simulink model "Joystick201401023GoldenTriangleLightTEST2"  (R2012b)
settings: Solver=ode4  StartTime=0.0  StopTime=inf  FixedStep=sample_time  RelTol=1e-3
InitFcn:
  | sample_time=0.005;%0.004;%0.0025;%0.02;
  | sample_time_Vicon = 0.005;
  | DeltaT = 0.02;
  | g = 9.81;
  | H0 = g%0.3165;
  | Kl = 1;
  | 
  | Omega_r = 1.31;%for Horizontal reference
  | Zeta_r = 1; %for Horizontal reference
  | Omega = 1.5;%1.31;%for Horizontal Control
  | Zeta = 0.5;    %for Horizontal Control
  | 
  | Omega_h_r = 2.2; %for vertical reference
  | Zeta_h_r = 1;  %for vertical reference
  | Omega_h = 2.2;    %for vertical control
  | Zeta_h = 1;         %for vertical control
  | PI=pi;
  | 
  | Mass = 1.1;
  | Acc_Max = 4;
  | Acc_Max_h = 4;
  | 
  | Max_RP = 60;
  | 
  | % for NN
  | n = 5;
  | r = 3;
  | n2 = 5;
  | NN_ST = 0.02;
  | 
  | GAMA_V = 3;
  | gama_V_e = 0.01;
  | 
  | GAMA_W = GAMA_V;
  | gama_W_e =0.01;
  | 
  | % deadzone
  | NN_Deadzone_Z = 0;
  | 
  | % inputs nomalizaton parameters
  | NN_Z_y_min = -3;
  | NN_Z_y_max = 0.5;
  | 
  | NN_Z_v_max = 8;
  | NN_Z_v_min = -NN_Z_v_max;
  | 
  | % alpha = 0.034;
  | alpha = 1;
  | % c_f = 0.0015;
  | c_f = 0.001;
  | c_y_tilt = 1*0.5;
  | 
  | %for WK paras
  | Heightcontrol = 0.08;
  | Scale_Factor=1;
  | yoffset=0;
  | 
  | load MaoBi_Oct04_2_int.mat
  | MB_Interp.time = [];
undefined symbols (not defined in the file or in its folder): DiscIntNeverNeededParam
libraries: simulink x8, X330_Control x4, vrlib x1
(part 1 of 2)
settings Model: Creator=ttcl3  LastModifiedBy=Vicon
settings SolverCC: MaxConsecutiveMinStep=auto
settings DataIOCC: SignalLoggingSaveFormat=ModelDataLogs
settings DebuggingCC: MultiTaskRateTransMsg=warning  FcnCallInpInsideContextMsg=UseLocalSettings
settings SFSimCC: SimParseCustomCode=off
settings GRTTargetCC: CombineOutputUpdateFcns=off  GRTInterface=on

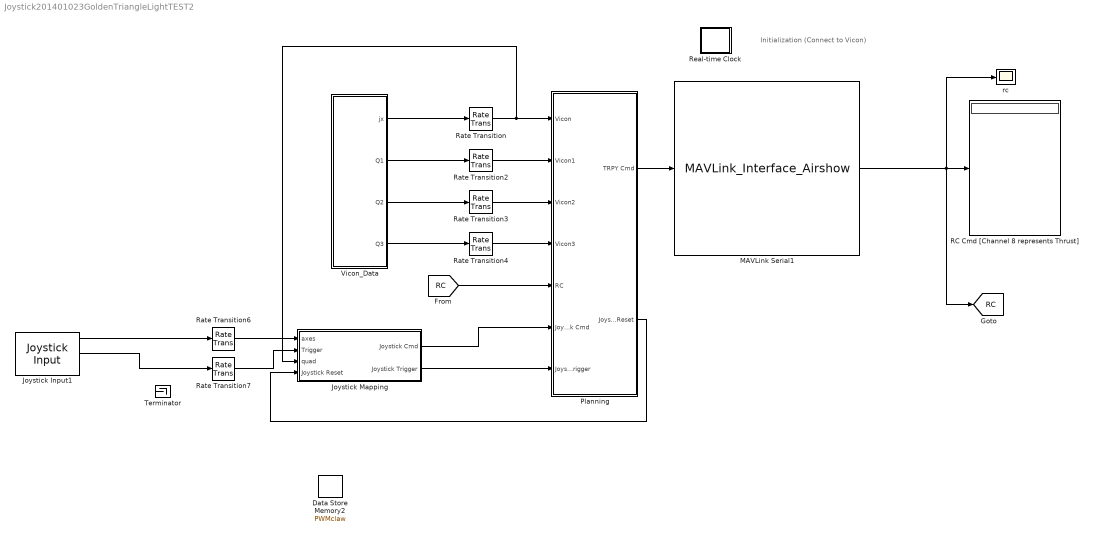
== system Joystick201401023GoldenTriangleLightTEST2 ==
  note: Initialization
      | (Connect to Vicon)
  Data Store Memory2 : DataStoreMemory  DataStoreName=PWMclaw  InitialValue=1690  OutDataTypeStr=double
  Joystick Input1 : vrlib/Joystick Input  joyid=1  adjustports=on  forcefeed=off
  Joystick Mapping : Subsystem
  MAVLink Serial1 : S-Function  FunctionName=MAVLink_Interface_Airshow  Parameters=COM_Port,Baud_Rate,MSG_INPUT,MSG_OUTPUT  EnableBusSupport=off  mask{COM_Port='COM2', Baud_Rate=57600, ATTITUDE_OUT=off, RC_SCALED=on, Quads_1=on, Quads_2=off, Quads_3=off, Quads_4=off, Quads_5=off, Quads_6=off}
      mask prompts: COM_Port "COM Port"; Baud_Rate "Baud Rate"; ATTITUDE_OUT "DEBUG"; RC_SCALED "RC CHANNELS SCALED"; Quads_1 "1 Quad"; Quads_2 "2 Quad"; Quads_3 "3 Quad"; Quads_4 "4 Quad"; Quads_5 "5 Quad"; Quads_6 "6 Quad"
      mask init:
      | MSG_ID_NUM_INPUT = [ uint8(221) uint8(222) uint8(223) uint8(224) uint8(225) uint8(226)];
      | MSG_ID_NAME_INPUT = [Quads_1 Quads_2 Quads_3 Quads_4 Quads_5 Quads_6];
      | 
      | MSG_ID_NUM_OUTPUT = [uint8(34) uint8(30)];
      | MSG_ID_NAME_OUTPUT = [RC_SCALED ATTITUDE_OUT ];
      | 
      | idx_input = find(MSG_ID_NAME_INPUT);
      | MSG_INPUT = MSG_ID_NUM_INPUT(idx_input);
      | 
      | idx_output = find(MSG_ID_NAME_OUTPUT);
      | MSG_OUTPUT = MSG_ID_NUM_OUTPUT(idx_output);
      mask Display:
      | % Block image
      | image(imread('10-inch Quad Heat Map.png'));
      | 
      | %Label block
      | fprintf('MAVLink Serial\n%s\n%dbps', COM_Port,  Baud_Rate)
      | 
      | 
      | %Label input ports
      | 
      | in = 1;
      | if (Quads_1 == 1)
      |     port_label('input', in, 'Quads_1');
      |     in = in + 1;
      | end
      | 
      | if (Quads_2 == 1)
      |     port_label('input', in, 'Quads_2');
      |     in = in + 1;
      | end
      | 
      | if (Quads_3 == 1)
      |     port_label('input', in, 'Quads_3');
      |     in = in + 1;
      | end
      | 
      | if (Quads_4 == 1)
      |     port_label('input', in, 'Quads_4');
      |     in = in + 1;
      | end
      | 
      | if (Quads_5 == 1)
      |     port_label('input', in, 'Quads_5');
      |     in = in + 1;
      | end
      | 
      | 
      | if (Quads_6 == 1)
      |     port_label('input', in, 'Quads_6');
      |     in = in + 1;
      | end
      | %Label output ports
      | 
      | out = 1;
      | if (RC_SCALED == 1)
      |     port_label('output', out, 'RC CMD');
      |     out = out + 1;
      | end
      | 
      | if (ATTITUDE_OUT == 1)
      |     port_label('output', out, 'DEBUG');
      |     out = out + 1;
      | end
  Planning : Subsystem
  RC Cmd [Channel 8 represents Thrust] : Display
  Rate Transition{,2..4,6..7} (6 alike) : RateTransition  OutPortSampleTime=0.02
  Real-time Clock : Subsystem  mask(Real-time Clock){sample_time=0.02, tolerance=1}
      mask prompts: sample_time "Synchronize with real-time every n seconds:"; tolerance "Real-time warning tolerance (seconds):"
      mask help: Real-time Synchronization Block
      mask Help: This block synchronizes simulation time with the PC real-time clock or UNIX system clock. The first dialog entry is the period at which the clock is checked to insure real-time synchronization. The second dialog entry is the number of seconds that the simulation time must be within real-time before a warning is printed.
      mask Display: plot(0,0,100,100,[40,60,60,54,54,64,69,76,82,77,81,83,83,81,78,74,70,64,57,49,41,35,32,30,30,31,34,40,47,47,40,40],[90,90,85,85,80,79,76,87,80,70,64,57,49,41,33,28,24,22,21,23,25,31,37,46,56,65,73,78,80,85,85,90],[69,53,53],[64,50,73])
  Terminator : Terminator
  Vicon_Data : Subsystem
  rc : Scope
      settings: TimeRange=10  YMin=-1  YMax=0.1
  tag scope: RC=global
  wires:
  [RC] -> Planning/5(RC)
  MAVLink Serial1/1 -> [RC], rc/1, RC Cmd [Channel 8 represents Thrust]/1
  Rate Transition/1 -> Joystick Mapping/3(quad), Planning/1(Vicon)
  Vicon_Data/4(Q3) -> Rate Transition4/1
  Vicon_Data/3(Q2) -> Rate Transition3/1
  Vicon_Data/2(Q1) -> Rate Transition2/1
  Rate Transition4/1 -> Planning/4(Vicon3)
  Rate Transition3/1 -> Planning/3(Vicon2)
  Rate Transition2/1 -> Planning/2(Vicon1)
  Planning/1(TRPY Cmd) -> MAVLink Serial1/1
  Joystick Input1/1 -> Rate Transition6/1
  Joystick Mapping/1(Joystick Cmd) -> Planning/6(Joystick Cmd)
  Rate Transition6/1 -> Joystick Mapping/1(axes)
  Rate Transition7/1 -> Joystick Mapping/2(Trigger)
  Vicon_Data/1(jx) -> Rate Transition/1
  Planning/2(JoystickReset) -> Joystick Mapping/4(Joystick Reset)
  Joystick Mapping/2(Joystick Trigger) -> Planning/7(Joystick Trigger)
  Joystick Input1/2 -> Rate Transition7/1
  ? -> Terminator/1

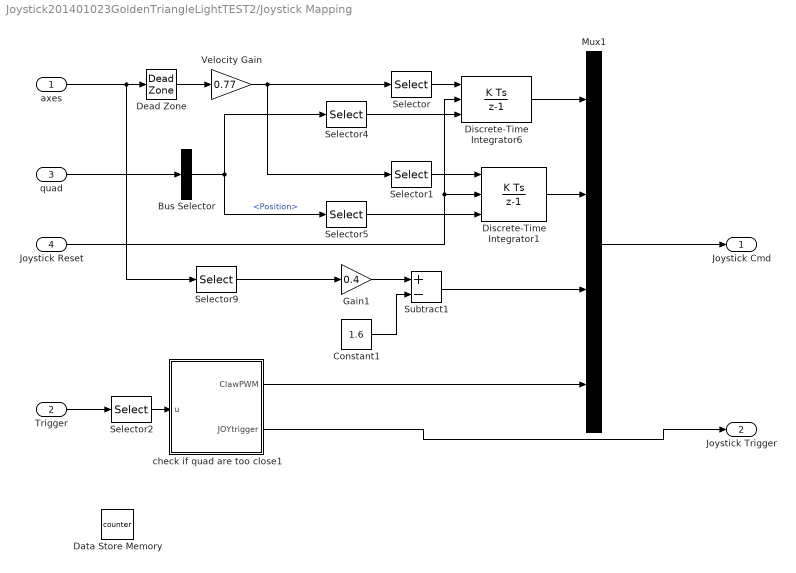
== system Joystick201401023GoldenTriangleLightTEST2/Joystick Mapping ==
  axes : Inport
  Trigger : Inport  Port=2
  quad : Inport  Port=3
  Joystick Reset : Inport  Port=4
  Bus Selector : BusSelector  OutputSignals=Position
  Constant1 : Constant  Value=1.6
  Data Store Memory : DataStoreMemory  DataStoreName=counter  InitialValue=25  OutDataTypeStr=double
  Dead Zone : DeadZone  LowerValue=-0.01  UpperValue=0.01  SaturateOnIntegerOverflow=on
  Discrete-Time Integrator1 : DiscreteIntegrator  gainval=1  ExternalReset=level  InitialConditionSource=external  SampleTime=0.02  OutMin=-3.5  OutMax=3.5  LimitOutput=on  UpperSaturationLimit=3.5  LowerSaturationLimit=-3.5  ICPrevOutput=DiscIntNeverNeededParam  ICPrevScaledInput=DiscIntNeverNeededParam
  Discrete-Time Integrator6 : DiscreteIntegrator  gainval=1  ExternalReset=level  InitialConditionSource=external  SampleTime=0.02  OutMin=-3.5  OutMax=3.5  LimitOutput=on  UpperSaturationLimit=3.5  LowerSaturationLimit=-3.5  ICPrevOutput=DiscIntNeverNeededParam  ICPrevScaledInput=DiscIntNeverNeededParam
  Gain1 : Gain  Gain=0.4
  Mux1 : Mux
  Selector : Selector  IndexOptions=Index vector (dialog)  Indices=[1]  OutputSizes=1
  Selector1 : Selector  IndexOptions=Index vector (dialog)  Indices=[2]  OutputSizes=1
  Selector2 : Selector  IndexOptions=Index vector (dialog)  Indices=[1]  OutputSizes=1
  Selector4 : Selector  InputPortWidth=3  IndexOptions=Index vector (dialog)  Indices=[1]  OutputSizes=1
  Selector5 : Selector  InputPortWidth=3  IndexOptions=Index vector (dialog)  Indices=[2]  OutputSizes=1
  Selector9 : Selector  IndexOptions=Index vector (dialog)  Indices=[3]  OutputSizes=1
  Subtract1 : Sum  Inputs=+-  OutMin=-2.5  OutMax=-1
  Velocity Gain : Gain  Gain=0.77
  check if quad are too close1 : MATLAB Function  TreatAsAtomicUnit=on
  Joystick Cmd : Outport
  Joystick Trigger : Outport  Port=2
  wires:
  Selector1/1 -> Discrete-Time Integrator1/1
  Selector/1 -> Discrete-Time Integrator6/1
  Velocity Gain/1 -> Selector1/1, Selector/1
  axes/1 -> Dead Zone/1, Selector9/1
  Discrete-Time Integrator6/1 -> Mux1/1
  Discrete-Time Integrator1/1 -> Mux1/2
  Mux1/1 -> Joystick Cmd/1
  check if quad are too close1/1(ClawPWM) -> Mux1/4
  Selector2/1 -> check if quad are too close1/1(u)
  Trigger/1 -> Selector2/1
  quad/1 -> Bus Selector/1
  Bus Selector/1 -> Selector4/1, Selector5/1  "<Position>"
  Selector4/1 -> Discrete-Time Integrator6/3
  Selector5/1 -> Discrete-Time Integrator1/3
  Joystick Reset/1 -> Discrete-Time Integrator1/2, Discrete-Time Integrator6/2
  check if quad are too close1/2(JOYtrigger) -> Joystick Trigger/1
  Constant1/1 -> Subtract1/2
  Selector9/1 -> Gain1/1
  Gain1/1 -> Subtract1/1
  Subtract1/1 -> Mux1/3
  Dead Zone/1 -> Velocity Gain/1

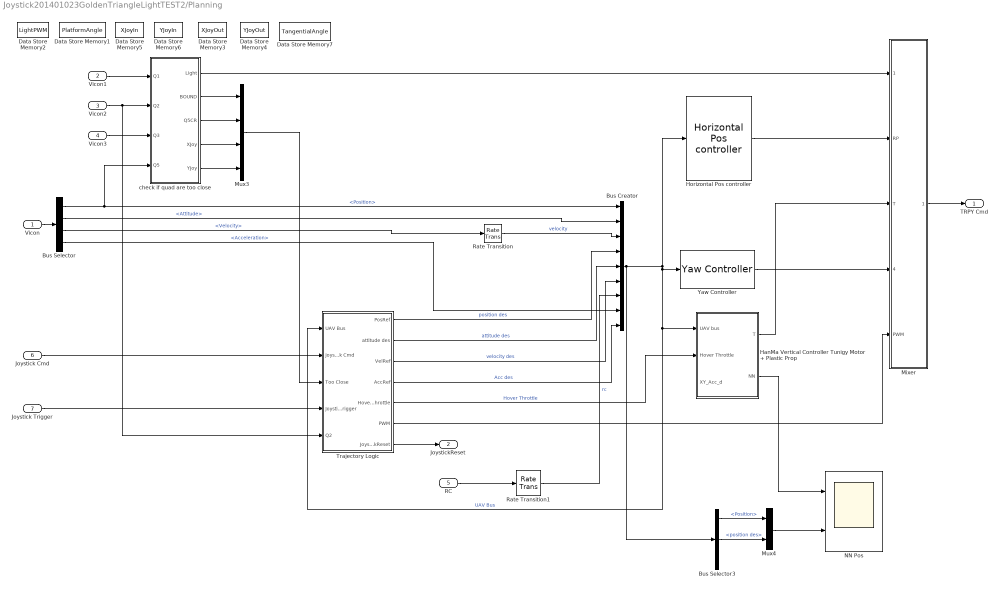
== system Joystick201401023GoldenTriangleLightTEST2/Planning ==
  Vicon : Inport
  Vicon1 : Inport  Port=2
  Vicon2 : Inport  Port=3
  Vicon3 : Inport  Port=4
  RC : Inport  Port=5
  Joystick Cmd : Inport  Port=6
  Joystick Trigger : Inport  Port=7
  Bus Creator : BusCreator  Inputs=9
  Bus Selector : BusSelector  OutputSignals=Position,Attitude,Velocity,Acceleration
  Bus Selector3 : BusSelector  OutputSignals=Position,position des,Attitude
  Data Store Memory1 : DataStoreMemory  DataStoreName=PlatformAngle  OutDataTypeStr=double
  Data Store Memory2 : DataStoreMemory  DataStoreName=LightPWM  OutMin=-3.3  OutMax=3.3  OutDataTypeStr=double
  Data Store Memory3 : DataStoreMemory  DataStoreName=XJoyOut  OutMin=-3.5  OutMax=3.5  OutDataTypeStr=double
  Data Store Memory4 : DataStoreMemory  DataStoreName=YJoyOut  OutMin=-3.5  OutMax=3.5  OutDataTypeStr=double
  Data Store Memory5 : DataStoreMemory  DataStoreName=XJoyIn  OutMin=-3.3  OutMax=3.3  OutDataTypeStr=double
  Data Store Memory6 : DataStoreMemory  DataStoreName=YJoyIn  OutMin=-3.3  OutMax=3.3  OutDataTypeStr=double
  Data Store Memory7 : DataStoreMemory  DataStoreName=TangentialAngle  OutDataTypeStr=double
  HanMa Vertical Controller Tunigy Motor + Plastic Prop : Subsystem  mask{Omega_h=Omega_h, Zeta_h=Zeta_h, PID_I_h=0, mass=1.1}
      mask prompts: Omega_h "Omega (P Gain  = Omega^2)"; Zeta_h "Zeta (D Gain = 2*Omega*Zeta)"; PID_I_h "I Gain"
  Horizontal Pos controller : X330_Control/Horizontal Pos controller  Max_RP=Max_RP  Omega=Omega  PID_i=0.5  Zeta=Zeta
      link override Horizontal Position Controller/Saturation1: UpperLimit=3.4  LowerLimit=-3.4
  Mixer : Subsystem
  Mux3 : Mux
  Mux4 : Mux  Inputs=2
  NN Pos : Scope  NumInputPorts=2
      settings: TimeRange=90  YMin=-1.25~-3  YMax=3.5~0  SaveName=ScopeData3
  Rate Transition : RateTransition  OutPortSampleTime=0.02
  Rate Transition1 : RateTransition  OutPortSampleTime=0.02
  Trajectory Logic : Subsystem
  Yaw Controller : X330_Control/Yaw Controller
  check if quad are too close : MATLAB Function  TreatAsAtomicUnit=on
  TRPY Cmd : Outport
  JoystickReset : Outport  Port=2
  wires:
  Horizontal Pos controller/1 -> Mixer/2(RP)
  Rate Transition/1 -> Bus Creator/3  "velocity"
  Rate Transition1/1 -> Bus Creator/7  "rc"
  Bus Creator/1 -> Yaw Controller/1, Trajectory Logic/1(UAV Bus), HanMa Vertical Controller Tunigy Motor + Plastic Prop/1(UAV bus), Horizontal Pos controller/1, Bus Selector3/1  "UAV Bus"
  Yaw Controller/1 -> Mixer/4(Yaw rate)
  HanMa Vertical Controller Tunigy Motor + Plastic Prop/1(T) -> Mixer/3(T)
  Bus Selector/4 -> Bus Creator/8  "<Acceleration>"
  Trajectory Logic/1(PosRef) -> Bus Creator/4  "position des"
  Trajectory Logic/2(attitude des) -> Bus Creator/5  "attitude des"
  Trajectory Logic/3(VelRef) -> Bus Creator/6  "velocity des"
  Trajectory Logic/5(HoverThrottle) -> HanMa Vertical Controller Tunigy Motor + Plastic Prop/2(Hover Throttle)  "Hover Throttle"
  Bus Selector/1 -> check if quad are too close/4(Q5), Bus Creator/1  "<Position>"
  Bus Selector/2 -> Bus Creator/2  "<Attitude>"
  Bus Selector/3 -> Rate Transition/1  "<Velocity>"
  Vicon/1 -> Bus Selector/1
  Mixer/1(XYZ RPY) -> TRPY Cmd/1
  Trajectory Logic/4(AccRef) -> Bus Creator/9  "Acc des"
  RC/1 -> Rate Transition1/1
  Trajectory Logic/6(PWM) -> Mixer/5(PWM)
  Mux4/1 -> NN Pos/2
  Bus Selector3/1 -> Mux4/1  "<Position>"
  Bus Selector3/2 -> Mux4/2  "<position des>"
  HanMa Vertical Controller Tunigy Motor + Plastic Prop/2(NN) -> NN Pos/1
  Joystick Cmd/1 -> Trajectory Logic/2(Joystick Cmd)
  Mux3/1 -> Trajectory Logic/3(Too Close)
  Vicon3/1 -> check if quad are too close/3(Q3)
  Vicon2/1 -> Trajectory Logic/5(Q2), check if quad are too close/2(Q2)
  Vicon1/1 -> check if quad are too close/1(Q1)
  Trajectory Logic/7(JoystickReset) -> JoystickReset/1
  check if quad are too close/2(BOUND) -> Mux3/1
  check if quad are too close/3(Q5CR) -> Mux3/2
  check if quad are too close/4(XJoy) -> Mux3/3
  check if quad are too close/5(YJoy) -> Mux3/4
  Joystick Trigger/1 -> Trajectory Logic/4(Joystick Trigger)
  check if quad are too close/1(Light) -> Mixer/1(Light PWM)

== system Joystick201401023GoldenTriangleLightTEST2/Real-time Clock ==
  Real-time Clock : S-Function  FunctionName=rtclock  Parameters=sample_time, tolerance  EnableBusSupport=off

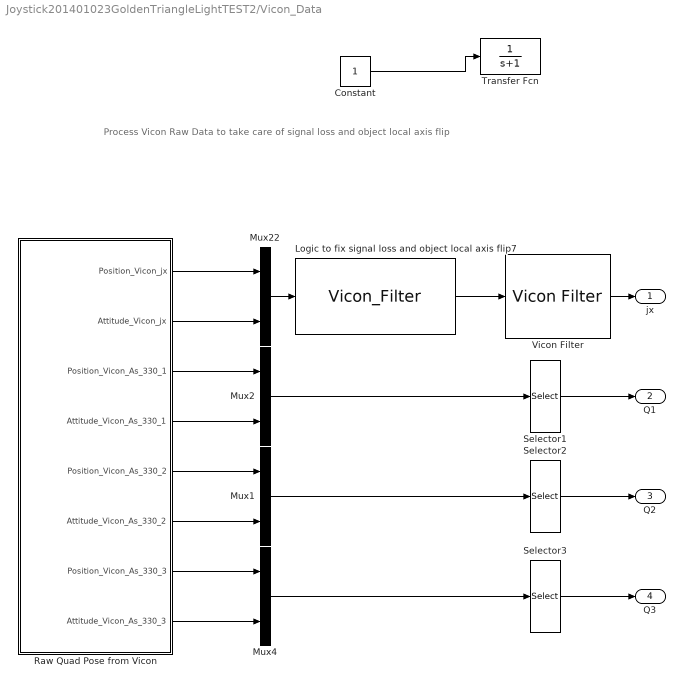
== system Joystick201401023GoldenTriangleLightTEST2/Vicon_Data ==
  note: Process Vicon Raw Data to take care of signal loss and object local axis flip
  Constant : Constant
  Logic to fix signal loss and object local axis flip7 : M-S-Function  FunctionName=Vicon_Filter
  Mux{1..2,4,22} (4 alike) : Mux  Inputs=2
  Raw Quad Pose from Vicon : Subsystem
  Selector1 : Selector  InputPortWidth=6  IndexOptions=Index vector (dialog)  Indices=[1 2]  OutputSizes=1
  Selector2 : Selector  InputPortWidth=6  IndexOptions=Index vector (dialog)  Indices=[1 2 3]  OutputSizes=1
  Selector3 : Selector  InputPortWidth=6  IndexOptions=Index vector (dialog)  Indices=[1 2]  OutputSizes=1
  Transfer Fcn : TransferFcn  Denominator=[1 1]
  Vicon Filter : X330_Control/Vicon Filter
  jx : Outport
  Q1 : Outport  Port=2
  Q2 : Outport  Port=3
  Q3 : Outport  Port=4
  wires:
  Raw Quad Pose from Vicon/2(Attitude_Vicon_jx) -> Mux22/2
  Raw Quad Pose from Vicon/1(Position_Vicon_jx) -> Mux22/1
  Logic to fix signal loss and object local axis flip7/1 -> Vicon Filter/1
  Mux2/1 -> Selector1/1
  Selector1/1 -> Q1/1
  Raw Quad Pose from Vicon/4(Attitude_Vicon_As_330_1) -> Mux2/2
  Raw Quad Pose from Vicon/3(Position_Vicon_As_330_1) -> Mux2/1
  Selector2/1 -> Q2/1
  Mux1/1 -> Selector2/1
  Raw Quad Pose from Vicon/5(Position_Vicon_As_330_2) -> Mux1/1
  Raw Quad Pose from Vicon/6(Attitude_Vicon_As_330_2) -> Mux1/2
  Mux4/1 -> Selector3/1
  Selector3/1 -> Q3/1
  Raw Quad Pose from Vicon/8(Attitude_Vicon_As_330_3) -> Mux4/2
  Raw Quad Pose from Vicon/7(Position_Vicon_As_330_3) -> Mux4/1
  Constant/1 -> Transfer Fcn/1
  Mux22/1 -> Logic to fix signal loss and object local axis flip7/1
  Vicon Filter/1 -> jx/1

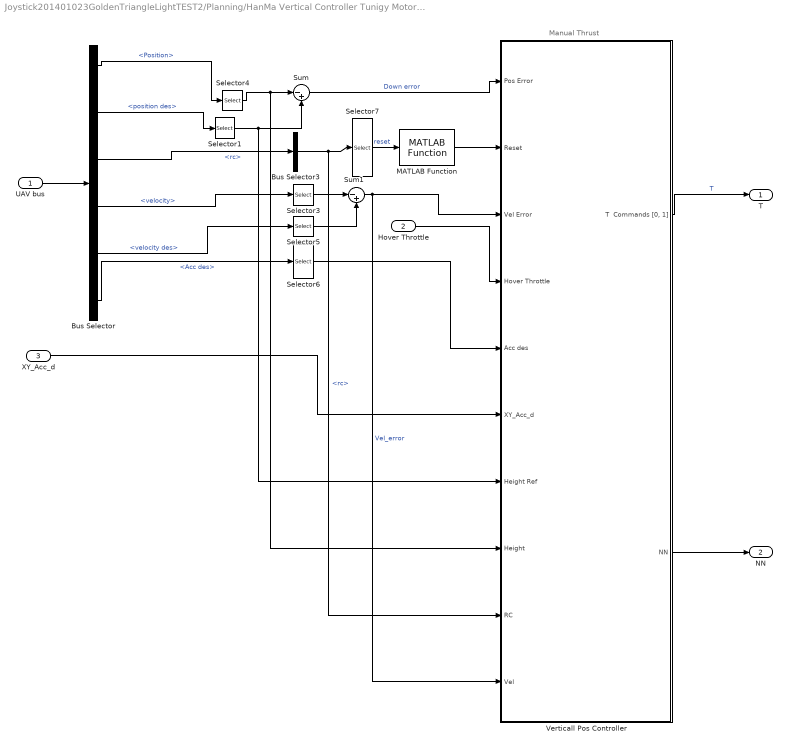
== system Joystick201401023GoldenTriangleLightTEST2/Planning/HanMa Vertical Controller Tunigy Motor + Plastic Prop ==
  note: Manual Thrust
  UAV bus : Inport
  Hover Throttle : Inport  Port=2
  XY_Acc_d : Inport  Port=3
  Bus Selector : BusSelector  OutputSignals=Position,position des,rc,velocity,velocity des,Acc des
  Bus Selector3 : BusSelector  OutputSignals=rc
  MATLAB Function : X330_Control/NN For Height AxiMotor + APC Prop/MATLAB Function
  Selector{1,3..5} (4 alike) : Selector  InputPortWidth=3  IndexOptions=Index vector (dialog)  Indices=[3]  OutputSizes=1
  Selector6 : Selector  InputPortWidth=4  IndexOptions=Index vector (dialog)  Indices=[3]  OutputSizes=1
  Selector7 : Selector  InputPortWidth=8  IndexOptions=Index vector (dialog)  Indices=[7]  OutputSizes=1
  Sum : Sum  Inputs=|-+
  Sum1 : Sum  Inputs=|-+
  Verticall Pos Controller : Subsystem
  T : Outport
  NN : Outport  Port=2
  wires:
  XY_Acc_d/1 -> Verticall Pos Controller/6(XY_Acc_d)
  Verticall Pos Controller/1("T  Commands [0, 1]") -> T/1  "T"
  Selector6/1 -> Verticall Pos Controller/5(Acc des)
  Bus Selector/6 -> Selector6/1  "<Acc des>"
  Hover Throttle/1 -> Verticall Pos Controller/4(Hover Throttle)
  Bus Selector/5 -> Selector5/1  "<velocity des>"
  Bus Selector/4 -> Selector3/1  "<velocity>"
  Selector5/1 -> Sum1/2
  Selector3/1 -> Sum1/1
  Sum1/1 -> Verticall Pos Controller/3(Vel Error), Verticall Pos Controller/10(Vel)  "Vel_error"
  Selector7/1 -> MATLAB Function/1  "reset"
  Bus Selector3/1 -> Selector7/1, Verticall Pos Controller/9(RC)  "<rc>"
  Selector1/1 -> Sum/2, Verticall Pos Controller/7(Height Ref)
  Selector4/1 -> Sum/1, Verticall Pos Controller/8(Height)
  Sum/1 -> Verticall Pos Controller/1(Pos Error)  "Down error"
  Bus Selector/2 -> Selector1/1  "<position des>"
  Bus Selector/1 -> Selector4/1  "<Position>"
  Bus Selector/3 -> Bus Selector3/1  "<rc>"
  UAV bus/1 -> Bus Selector/1
  Verticall Pos Controller/2(NN) -> NN/1
  MATLAB Function/1 -> Verticall Pos Controller/2(Reset)

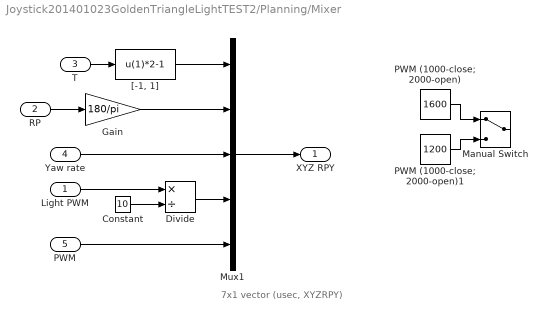
== system Joystick201401023GoldenTriangleLightTEST2/Planning/Mixer ==
  note: 7x1 vector (usec, XYZRPY)
  Light PWM : Inport
  RP : Inport  Port=2
  T : Inport  Port=3
  Yaw rate : Inport  Port=4
  PWM : Inport  Port=5
  Constant : Constant  Value=10
  Divide : Product  Inputs=*/
  Gain : Gain  Gain=180/pi
  Manual Switch : ManualSwitch
  Mux1 : Mux  Inputs=5
  PWM (1000-close; 2000-open) : Constant  Value=1600  SampleTime=0.02
  PWM (1000-close; 2000-open)1 : Constant  Value=1200  SampleTime=0.02
  "[-1, 1]" : Fcn  Expr=u(1)*2-1
  XYZ RPY : Outport
  wires:
  Mux1/1 -> XYZ RPY/1
  T/1 -> "[-1, 1]"/1
  RP/1 -> Gain/1
  PWM (1000-close; 2000-open)/1 -> Manual Switch/1
  PWM (1000-close; 2000-open)1/1 -> Manual Switch/2
  Gain/1 -> Mux1/2
  "[-1, 1]"/1 -> Mux1/1
  PWM/1 -> Mux1/5
  Constant/1 -> Divide/2
  Yaw rate/1 -> Mux1/3
  Divide/1 -> Mux1/4
  Light PWM/1 -> Divide/1

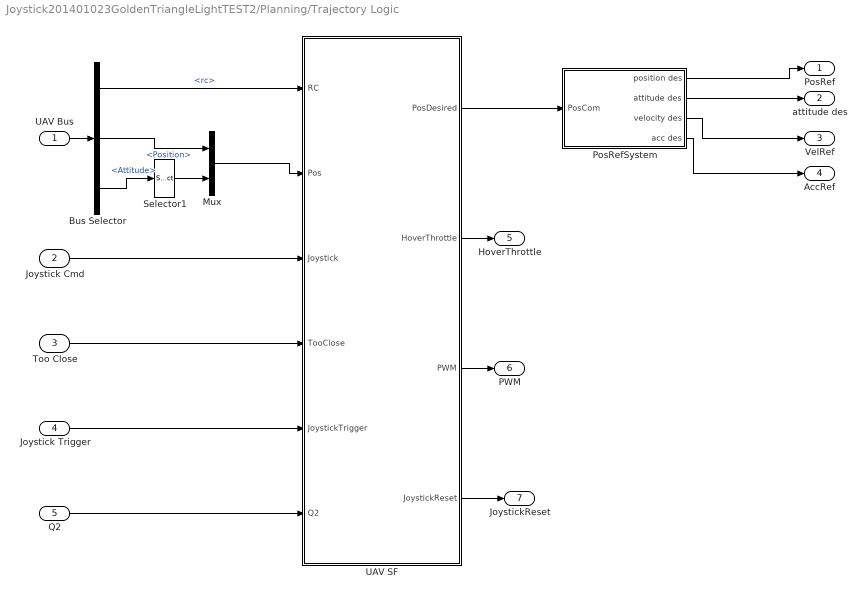
== system Joystick201401023GoldenTriangleLightTEST2/Planning/Trajectory Logic ==
  UAV Bus : Inport
  Joystick Cmd : Inport  Port=2
  Too Close : Inport  Port=3
  Joystick Trigger : Inport  Port=4
  Q2 : Inport  Port=5
  Bus Selector : BusSelector  OutputSignals=rc,Position,Attitude
  Mux : Mux  Inputs=2
  PosRefSystem : Subsystem  AncestorBlock=X330_Control/PosRefSystem  mask{Omega_r=Omega_r, Zeta_r=Zeta_r, Acc_Max=Acc_Max, Omega_h_r=Omega_h_r, Zeta_h_r=Zeta_h_r, Acc_h_Max=Acc_Max_h}
      mask prompts: Omega_r "Omega_r (P Gain= Omega_r^2)"; Zeta_r "Zeta_r (D = 2*Omega_r*Zeta_r)"
  Selector1 : Selector  InputPortWidth=3  IndexOptions=Index vector (dialog)  Indices=[3]  OutputSizes=1
  UAV SF : Stateflow chart  TreatAsAtomicUnit=on
  PosRef : Outport
  attitude des : Outport  Port=2
  VelRef : Outport  Port=3
  AccRef : Outport  Port=4
  HoverThrottle : Outport  Port=5
  PWM : Outport  Port=6
  JoystickReset : Outport  Port=7
  wires:
  UAV SF/1(PosDesired) -> PosRefSystem/1(PosCom)
  Bus Selector/1 -> UAV SF/1(RC)  "<rc>"
  UAV SF/2(HoverThrottle) -> HoverThrottle/1
  UAV Bus/1 -> Bus Selector/1
  Bus Selector/2 -> Mux/1  "<Position>"
  Bus Selector/3 -> Selector1/1  "<Attitude>"
  Selector1/1 -> Mux/2
  Mux/1 -> UAV SF/2(Pos)
  UAV SF/3(PWM) -> PWM/1
  PosRefSystem/1(position des) -> PosRef/1
  PosRefSystem/3(velocity des) -> VelRef/1
  PosRefSystem/4(acc des) -> AccRef/1
  PosRefSystem/2(attitude des) -> attitude des/1
  Joystick Cmd/1 -> UAV SF/3(Joystick)
  Too Close/1 -> UAV SF/4(TooClose)
  UAV SF/4(JoystickReset) -> JoystickReset/1
  Joystick Trigger/1 -> UAV SF/5(JoystickTrigger)
  Q2/1 -> UAV SF/6(Q2)

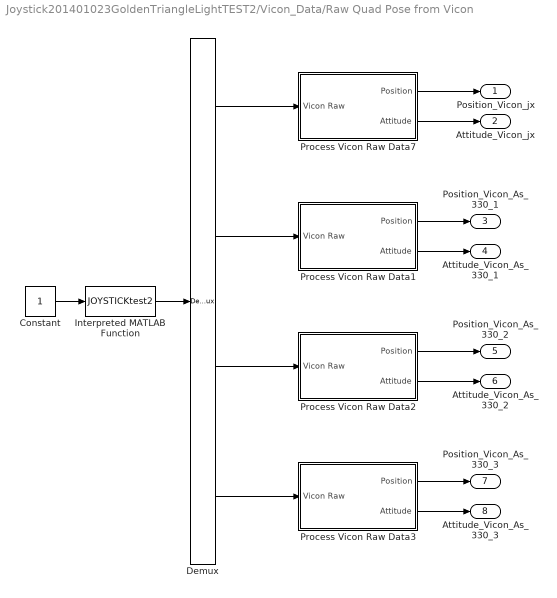
== system Joystick201401023GoldenTriangleLightTEST2/Vicon_Data/Raw Quad Pose from Vicon ==
  Constant : Constant
  Demux : Demux
  Interpreted MATLAB Function : MATLABFcn  MATLABFcn=JOYSTICKtest2  SampleTime=0.005
  Process Vicon Raw Data1 : Subsystem
  Process Vicon Raw Data2 : Subsystem
  Process Vicon Raw Data3 : Subsystem
  Process Vicon Raw Data7 : Subsystem
  Position_Vicon_jx : Outport
  Attitude_Vicon_jx : Outport  Port=2
  Position_Vicon_As_330_1 : Outport  Port=3
  Attitude_Vicon_As_330_1 : Outport  Port=4
  Position_Vicon_As_330_2 : Outport  Port=5
  Attitude_Vicon_As_330_2 : Outport  Port=6
  Position_Vicon_As_330_3 : Outport  Port=7
  Attitude_Vicon_As_330_3 : Outport  Port=8
  wires:
  Process Vicon Raw Data7/1(Position) -> Position_Vicon_jx/1
  Process Vicon Raw Data7/2(Attitude) -> Attitude_Vicon_jx/1
  Constant/1 -> Interpreted MATLAB Function/1
  Interpreted MATLAB Function/1 -> Demux/1
  Process Vicon Raw Data1/1(Position) -> Position_Vicon_As_330_1/1
  Process Vicon Raw Data1/2(Attitude) -> Attitude_Vicon_As_330_1/1
  Process Vicon Raw Data2/1(Position) -> Position_Vicon_As_330_2/1
  Process Vicon Raw Data2/2(Attitude) -> Attitude_Vicon_As_330_2/1
  Process Vicon Raw Data3/1(Position) -> Position_Vicon_As_330_3/1
  Process Vicon Raw Data3/2(Attitude) -> Attitude_Vicon_As_330_3/1
  Demux/1 -> Process Vicon Raw Data7/1(Vicon Raw)
  Demux/2 -> Process Vicon Raw Data1/1(Vicon Raw)
  Demux/3 -> Process Vicon Raw Data2/1(Vicon Raw)
  Demux/4 -> Process Vicon Raw Data3/1(Vicon Raw)

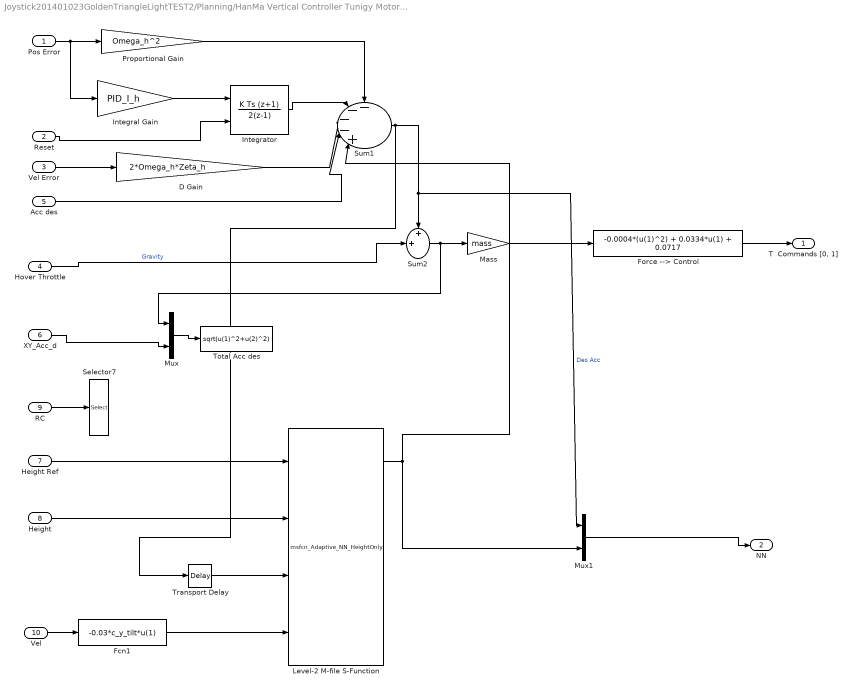
== system Joystick201401023GoldenTriangleLightTEST2/Planning/HanMa Vertical Controller Tunigy Motor + Plastic Prop/Verticall Pos Controller ==
  Pos Error : Inport
  Reset : Inport  Port=2
  Vel Error : Inport  Port=3
  Hover Throttle : Inport  Port=4
  Acc des : Inport  Port=5
  XY_Acc_d : Inport  Port=6
  Height Ref : Inport  Port=7
  Height : Inport  Port=8
  RC : Inport  Port=9
  Vel : Inport  Port=10
  D Gain : Gain  Gain=2*Omega_h*Zeta_h  OutDataTypeStr=double
  Fcn1 : Fcn  Expr=-0.03*c_y_tilt*u(1)
  Force --> Control : Fcn  Expr=-0.0004*(u(1)^2) + 0.0334*u(1) + 0.0717
  Integral Gain : Gain  DisableCoverage=on  Gain=PID_I_h  ParamDataTypeStr=double  OutDataTypeStr=double
  Integrator : DiscreteIntegrator  DisableCoverage=on  IntegratorMethod=Integration: Trapezoidal  ExternalReset=level  InitialConditionMode=State only (most efficient)  SampleTime=-1  OutDataTypeStr=double  UpperSaturationLimit=0.3  LowerSaturationLimit=-0.3  ICPrevOutput=DiscIntNeverNeededParam  ICPrevScaledInput=DiscIntNeverNeededParam
  Level-2 M-file S-Function : M-S-Function  FunctionName=msfcn_Adaptive_NN_HeightOnly  Parameters=n,r,n2,NN_ST,GAMA_V,gama_V_e,GAMA_W,gama_W_e,alpha,c_f,c_y_tilt,NN_Deadzone_Z,NN_Z_y_min,NN_Z_y_max,NN_Z_v_min,NN_Z_v_max
      mask Display: fprintf('Output Feedback NN \n Control Block')
  Mass : Gain  DisableCoverage=on  Gain=mass  ParamDataTypeStr=double  OutDataTypeStr=double
  Mux : Mux  Inputs=2
  Mux1 : Mux  Inputs=2
  Proportional Gain : Gain  DisableCoverage=on  Gain=Omega_h^2  ParamDataTypeStr=double  OutDataTypeStr=double
  Selector7 : Selector  InputPortWidth=8  IndexOptions=Index vector (dialog)  Indices=[6]  OutputSizes=1
  Sum1 : Sum  DisableCoverage=on  Inputs=----+|  AccumDataTypeStr=double  OutDataTypeStr=double  SampleTime=0.02
  Sum2 : Sum  DisableCoverage=on  Inputs=++|  AccumDataTypeStr=double  OutDataTypeStr=double  SampleTime=0.02
  Total Acc des : Fcn  Expr=sqrt(u(1)^2+u(2)^2)
  Transport Delay : TransportDelay  DelayTime=0.02
  "T  Commands [0, 1]" : Outport
  NN : Outport  Port=2
  wires:
  Force --> Control/1 -> "T  Commands [0, 1]"/1
  Sum2/1 -> Mux/1, Mass/1
  XY_Acc_d/1 -> Mux/2
  Mux/1 -> Total Acc des/1
  Mass/1 -> Force --> Control/1
  Sum1/1 -> Transport Delay/1, Sum2/1, Mux1/1  "Des Acc"
  Hover Throttle/1 -> Sum2/2  "Gravity"
  Acc des/1 -> Sum1/4
  D Gain/1 -> Sum1/3
  Vel Error/1 -> D Gain/1
  Reset/1 -> Integrator/2
  Pos Error/1 -> Integral Gain/1, Proportional Gain/1
  Proportional Gain/1 -> Sum1/1
  Integrator/1 -> Sum1/2
  Integral Gain/1 -> Integrator/1
  Height Ref/1 -> Level-2 M-file S-Function/1
  Level-2 M-file S-Function/1 -> Mux1/2, Sum1/5
  RC/1 -> Selector7/1
  Fcn1/1 -> Level-2 M-file S-Function/4
  Transport Delay/1 -> Level-2 M-file S-Function/3
  Mux1/1 -> NN/1
  Vel/1 -> Fcn1/1
  Height/1 -> Level-2 M-file S-Function/2

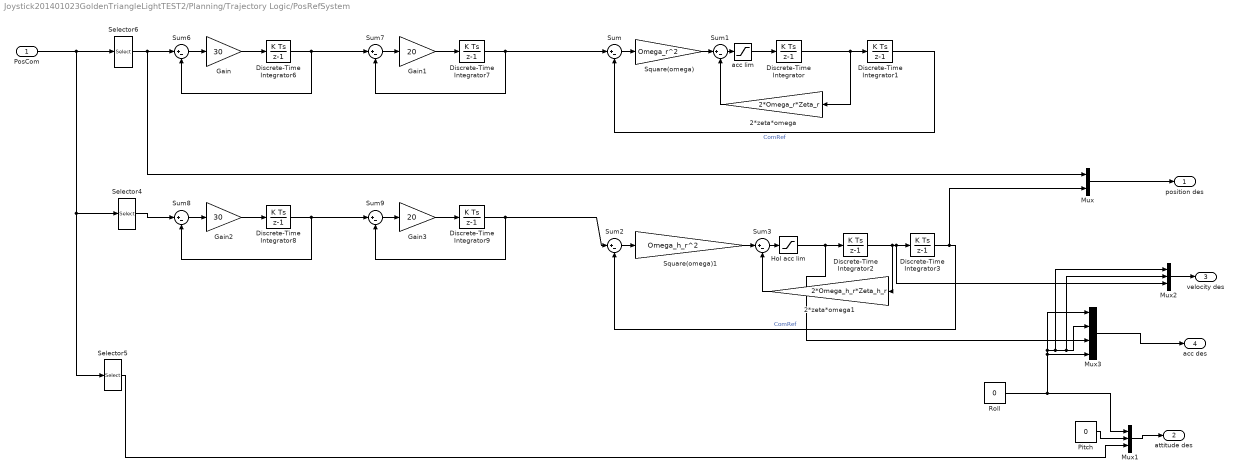
== system Joystick201401023GoldenTriangleLightTEST2/Planning/Trajectory Logic/PosRefSystem ==
  PosCom : Inport
  2*zeta*omega : Gain  Gain=2*Omega_r*Zeta_r
  2*zeta*omega1 : Gain  Gain=2*Omega_h_r*Zeta_h_r
  Discrete-Time Integrator{,1..3,6..9} (8 alike) : DiscreteIntegrator  SampleTime=-1  ICPrevOutput=DiscIntNeverNeededParam  ICPrevScaledInput=DiscIntNeverNeededParam
  Gain : Gain  Gain=30
  Gain1 : Gain  Gain=20
  Gain2 : Gain  Gain=30
  Gain3 : Gain  Gain=20
  Hol acc lim : Saturate  UpperLimit=Acc_h_Max  LowerLimit=-Acc_h_Max
  Mux : Mux  Inputs=2
  Mux1 : Mux  Inputs=3
  Mux2 : Mux  Inputs=3
  Mux3 : Mux
  Pitch : Constant  Value=0  SampleTime=0.02
  Roll : Constant  Value=0  SampleTime=0.02
  Selector4 : Selector  InputPortWidth=4  IndexOptions=Index vector (dialog)  Indices=[3]  OutputSizes=1
  Selector5 : Selector  InputPortWidth=4  IndexOptions=Index vector (dialog)  Indices=[4]  OutputSizes=1
  Selector6 : Selector  InputPortWidth=4  IndexOptions=Index vector (dialog)  Indices=[1 2]  OutputSizes=1
  Square(omega) : Gain  Gain=Omega_r^2
  Square(omega)1 : Gain  Gain=Omega_h_r^2
  Sum{,1..3,6..9} (8 alike) : Sum  Inputs=|+-
  acc lim : Saturate  UpperLimit=Acc_Max  LowerLimit=-Acc_Max
  position des : Outport
  attitude des : Outport  Port=2
  velocity des : Outport  Port=3
  acc des : Outport  Port=4
  wires:
  Sum9/1 -> Gain3/1
  Gain3/1 -> Discrete-Time Integrator9/1
  Discrete-Time Integrator9/1 -> Sum2/1, Sum9/2
  Sum8/1 -> Gain2/1
  Gain2/1 -> Discrete-Time Integrator8/1
  Discrete-Time Integrator8/1 -> Sum9/1, Sum8/2
  Selector4/1 -> Sum8/1
  Sum7/1 -> Gain1/1
  Gain1/1 -> Discrete-Time Integrator7/1
  Discrete-Time Integrator7/1 -> Sum/1, Sum7/2
  Sum6/1 -> Gain/1
  Gain/1 -> Discrete-Time Integrator6/1
  Discrete-Time Integrator6/1 -> Sum7/1, Sum6/2
  Selector6/1 -> Sum6/1, Mux/1
  Mux3/1 -> acc des/1
  Mux2/1 -> velocity des/1
  Mux1/1 -> attitude des/1
  Pitch/1 -> Mux1/2
  Roll/1 -> Mux3/2, Mux2/2, Mux2/1, Mux3/1, Mux3/4, Mux1/1
  Mux/1 -> position des/1
  Discrete-Time Integrator1/1 -> Sum/2  "ComRef"
  Hol acc lim/1 -> Mux3/3, Discrete-Time Integrator2/1
  2*zeta*omega1/1 -> Sum3/2
  Sum3/1 -> Hol acc lim/1
  Discrete-Time Integrator2/1 -> Mux2/3, Discrete-Time Integrator3/1, 2*zeta*omega1/1
  Square(omega)1/1 -> Sum3/1
  Sum2/1 -> Square(omega)1/1
  Discrete-Time Integrator3/1 -> Mux/2, Sum2/2  "ComRef"
  acc lim/1 -> Discrete-Time Integrator/1
  2*zeta*omega/1 -> Sum1/2
  Sum1/1 -> acc lim/1
  Discrete-Time Integrator/1 -> 2*zeta*omega/1, Discrete-Time Integrator1/1
  Square(omega)/1 -> Sum1/1
  Sum/1 -> Square(omega)/1
  PosCom/1 -> Selector6/1, Selector5/1, Selector4/1
  Selector5/1 -> Mux1/3

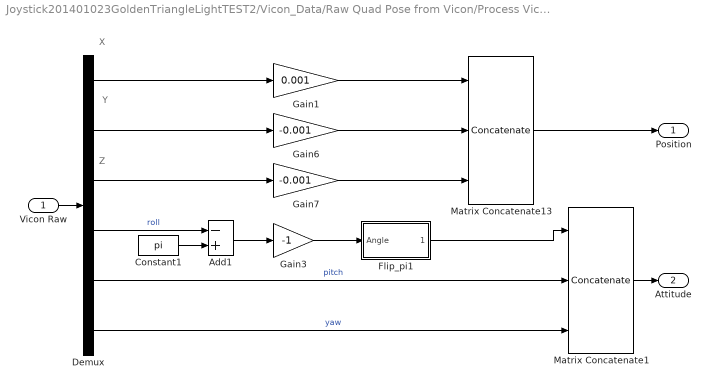
== system Joystick201401023GoldenTriangleLightTEST2/Vicon_Data/Raw Quad Pose from Vicon/Process Vicon Raw Data1 ==
  note: Z
  note: Y
  note: X
  Vicon Raw : Inport
  Add1 : Sum  Inputs=-+
  Constant1 : Constant  Value=pi  OutDataTypeStr=double
  Demux : Demux  Outputs=6
  Flip_pi1 : Subsystem  mask(Flip -pi to pi){}
      mask help: Flips the inputs into the range -pi to pi
      mask Help: Flips the inputs into the range -pi to pi
      mask Display: disp('Flip_pi')
  Gain1 : Gain  Gain=0.001
  Gain3 : Gain  Gain=-1
  Gain6 : Gain  Gain=-0.001
  Gain7 : Gain  Gain=-0.001
  Matrix Concatenate1 : Concatenate  NumInputs=3  Mode=Multidimensional array
  Matrix Concatenate13 : Concatenate  NumInputs=3  Mode=Multidimensional array
  Position : Outport
  Attitude : Outport  Port=2
  wires:
  Matrix Concatenate1/1 -> Attitude/1
  Vicon Raw/1 -> Demux/1
  Matrix Concatenate13/1 -> Position/1
  Flip_pi1/1(Angle_Flip) -> Matrix Concatenate1/1
  Demux/5 -> Matrix Concatenate1/2  "pitch"
  Gain3/1 -> Flip_pi1/1(Angle)
  Add1/1 -> Gain3/1
  Gain7/1 -> Matrix Concatenate13/3
  Gain6/1 -> Matrix Concatenate13/2
  Demux/4 -> Add1/1  "roll"
  Demux/3 -> Gain7/1
  Demux/2 -> Gain6/1
  Demux/1 -> Gain1/1
  Gain1/1 -> Matrix Concatenate13/1
  Demux/6 -> Matrix Concatenate1/3  "yaw"
  Constant1/1 -> Add1/2

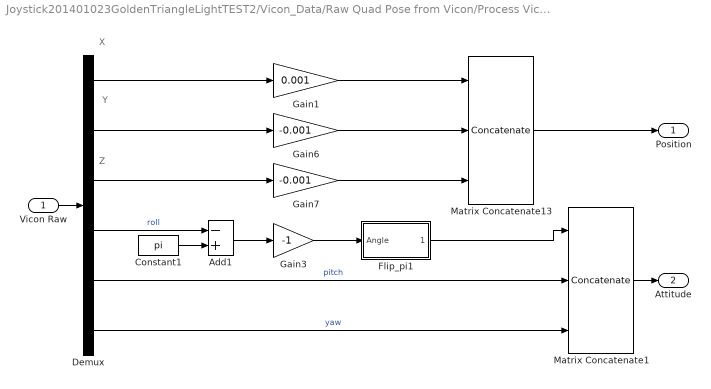
== system Joystick201401023GoldenTriangleLightTEST2/Vicon_Data/Raw Quad Pose from Vicon/Process Vicon Raw Data2 ==
  note: X
  note: Y
  note: Z
  Vicon Raw : Inport
  Add1 : Sum  Inputs=-+
  Constant1 : Constant  Value=pi  OutDataTypeStr=double
  Demux : Demux  Outputs=6
  Flip_pi1 : Subsystem  mask(Flip -pi to pi){}
      mask help: Flips the inputs into the range -pi to pi
      mask Help: Flips the inputs into the range -pi to pi
      mask Display: disp('Flip_pi')
  Gain1 : Gain  Gain=0.001
  Gain3 : Gain  Gain=-1
  Gain6 : Gain  Gain=-0.001
  Gain7 : Gain  Gain=-0.001
  Matrix Concatenate1 : Concatenate  NumInputs=3  Mode=Multidimensional array
  Matrix Concatenate13 : Concatenate  NumInputs=3  Mode=Multidimensional array
  Position : Outport
  Attitude : Outport  Port=2
  wires:
  Constant1/1 -> Add1/2
  Demux/6 -> Matrix Concatenate1/3  "yaw"
  Gain1/1 -> Matrix Concatenate13/1
  Demux/1 -> Gain1/1
  Demux/2 -> Gain6/1
  Demux/3 -> Gain7/1
  Demux/4 -> Add1/1  "roll"
  Gain6/1 -> Matrix Concatenate13/2
  Gain7/1 -> Matrix Concatenate13/3
  Add1/1 -> Gain3/1
  Gain3/1 -> Flip_pi1/1(Angle)
  Demux/5 -> Matrix Concatenate1/2  "pitch"
  Flip_pi1/1(Angle_Flip) -> Matrix Concatenate1/1
  Matrix Concatenate13/1 -> Position/1
  Vicon Raw/1 -> Demux/1
  Matrix Concatenate1/1 -> Attitude/1

== system Joystick201401023GoldenTriangleLightTEST2/Vicon_Data/Raw Quad Pose from Vicon/Process Vicon Raw Data3 ==
  note: Z
  note: Y
  note: X
  Vicon Raw : Inport
  Add1 : Sum  Inputs=-+
  Constant1 : Constant  Value=pi  OutDataTypeStr=double
  Demux : Demux  Outputs=6
  Flip_pi1 : Subsystem  mask(Flip -pi to pi){}
      mask help: Flips the inputs into the range -pi to pi
      mask Help: Flips the inputs into the range -pi to pi
      mask Display: disp('Flip_pi')
  Gain1 : Gain  Gain=0.001
  Gain3 : Gain  Gain=-1
  Gain6 : Gain  Gain=-0.001
  Gain7 : Gain  Gain=-0.001
  Matrix Concatenate1 : Concatenate  NumInputs=3  Mode=Multidimensional array
  Matrix Concatenate13 : Concatenate  NumInputs=3  Mode=Multidimensional array
  Position : Outport
  Attitude : Outport  Port=2
  wires:
  Matrix Concatenate1/1 -> Attitude/1
  Vicon Raw/1 -> Demux/1
  Matrix Concatenate13/1 -> Position/1
  Flip_pi1/1(Angle_Flip) -> Matrix Concatenate1/1
  Demux/5 -> Matrix Concatenate1/2  "pitch"
  Gain3/1 -> Flip_pi1/1(Angle)
  Add1/1 -> Gain3/1
  Gain7/1 -> Matrix Concatenate13/3
  Gain6/1 -> Matrix Concatenate13/2
  Demux/4 -> Add1/1  "roll"
  Demux/3 -> Gain7/1
  Demux/2 -> Gain6/1
  Demux/1 -> Gain1/1
  Gain1/1 -> Matrix Concatenate13/1
  Demux/6 -> Matrix Concatenate1/3  "yaw"
  Constant1/1 -> Add1/2

== system Joystick201401023GoldenTriangleLightTEST2/Vicon_Data/Raw Quad Pose from Vicon/Process Vicon Raw Data7 ==
  note: X
  note: Y
  note: Z
  Vicon Raw : Inport
  Add1 : Sum  Inputs=-+
  Constant1 : Constant  Value=pi  OutDataTypeStr=double
  Demux : Demux  Outputs=6
  Flip_pi1 : Subsystem  mask(Flip -pi to pi){}
      mask help: Flips the inputs into the range -pi to pi
      mask Help: Flips the inputs into the range -pi to pi
      mask Display: disp('Flip_pi')
  Gain1 : Gain  Gain=0.001
  Gain3 : Gain  Gain=-1
  Gain6 : Gain  Gain=-0.001
  Gain7 : Gain  Gain=-0.001
  Matrix Concatenate1 : Concatenate  NumInputs=3  Mode=Multidimensional array
  Matrix Concatenate13 : Concatenate  NumInputs=3  Mode=Multidimensional array
  Position : Outport
  Attitude : Outport  Port=2
  wires:
  Constant1/1 -> Add1/2
  Demux/6 -> Matrix Concatenate1/3  "yaw"
  Gain1/1 -> Matrix Concatenate13/1
  Demux/1 -> Gain1/1
  Demux/2 -> Gain6/1
  Demux/3 -> Gain7/1
  Demux/4 -> Add1/1  "roll"
  Gain6/1 -> Matrix Concatenate13/2
  Gain7/1 -> Matrix Concatenate13/3
  Add1/1 -> Gain3/1
  Gain3/1 -> Flip_pi1/1(Angle)
  Demux/5 -> Matrix Concatenate1/2  "pitch"
  Flip_pi1/1(Angle_Flip) -> Matrix Concatenate1/1
  Matrix Concatenate13/1 -> Position/1
  Vicon Raw/1 -> Demux/1
  Matrix Concatenate1/1 -> Attitude/1

== system Joystick201401023GoldenTriangleLightTEST2/Vicon_Data/Raw Quad Pose from Vicon/Process Vicon Raw Data1/Flip_pi1 ==
  Angle : Inport
  Add : Sum  Inputs=-+
  Compare To Constant1 : simulink/Logic and Bit Operations/Compare To Constant  relop=>  const=pi  OutDataTypeStr=uint8  ZeroCross=off
  Constant : Constant  Value=2*pi
  Data Type Duplicate : DataTypeDuplicate
  Flip_0_to_2pi : Subsystem  mask(Flip zero to 2pi){}
      mask help: Flips the inputs into the range zero to +2pi
      mask Help: Flips the inputs into the range zero to +2pi
      mask Display: disp('Flip_0_2pi')
  Switch : Switch  Criteria=u2 ~= 0
  Angle_Flip : Outport
  wires:
  Angle/1 -> Flip_0_to_2pi/1(Angle), Data Type Duplicate/2
  Flip_0_to_2pi/1(Angle_Flip) -> Switch/3, Compare To Constant1/1, Add/2
  Compare To Constant1/1 -> Switch/2
  Constant/1 -> Add/1
  Add/1 -> Switch/1
  Switch/1 -> Angle_Flip/1, Data Type Duplicate/1

== system Joystick201401023GoldenTriangleLightTEST2/Vicon_Data/Raw Quad Pose from Vicon/Process Vicon Raw Data2/Flip_pi1 ==
  Angle : Inport
  Add : Sum  Inputs=-+
  Compare To Constant1 : simulink/Logic and Bit Operations/Compare To Constant  relop=>  const=pi  OutDataTypeStr=uint8  ZeroCross=off
  Constant : Constant  Value=2*pi
  Data Type Duplicate : DataTypeDuplicate
  Flip_0_to_2pi : Subsystem  mask(Flip zero to 2pi){}
      mask help: Flips the inputs into the range zero to +2pi
      mask Help: Flips the inputs into the range zero to +2pi
      mask Display: disp('Flip_0_2pi')
  Switch : Switch  Criteria=u2 ~= 0
  Angle_Flip : Outport
  wires:
  Switch/1 -> Data Type Duplicate/1, Angle_Flip/1
  Add/1 -> Switch/1
  Constant/1 -> Add/1
  Compare To Constant1/1 -> Switch/2
  Flip_0_to_2pi/1(Angle_Flip) -> Add/2, Compare To Constant1/1, Switch/3
  Angle/1 -> Data Type Duplicate/2, Flip_0_to_2pi/1(Angle)

== system Joystick201401023GoldenTriangleLightTEST2/Vicon_Data/Raw Quad Pose from Vicon/Process Vicon Raw Data3/Flip_pi1 ==
  Angle : Inport
  Add : Sum  Inputs=-+
  Compare To Constant1 : simulink/Logic and Bit Operations/Compare To Constant  relop=>  const=pi  OutDataTypeStr=uint8  ZeroCross=off
  Constant : Constant  Value=2*pi
  Data Type Duplicate : DataTypeDuplicate
  Flip_0_to_2pi : Subsystem  mask(Flip zero to 2pi){}
      mask help: Flips the inputs into the range zero to +2pi
      mask Help: Flips the inputs into the range zero to +2pi
      mask Display: disp('Flip_0_2pi')
  Switch : Switch  Criteria=u2 ~= 0
  Angle_Flip : Outport
  wires:
  Angle/1 -> Flip_0_to_2pi/1(Angle), Data Type Duplicate/2
  Flip_0_to_2pi/1(Angle_Flip) -> Switch/3, Compare To Constant1/1, Add/2
  Compare To Constant1/1 -> Switch/2
  Constant/1 -> Add/1
  Add/1 -> Switch/1
  Switch/1 -> Angle_Flip/1, Data Type Duplicate/1

== system Joystick201401023GoldenTriangleLightTEST2/Vicon_Data/Raw Quad Pose from Vicon/Process Vicon Raw Data7/Flip_pi1 ==
  Angle : Inport
  Add : Sum  Inputs=-+
  Compare To Constant1 : simulink/Logic and Bit Operations/Compare To Constant  relop=>  const=pi  OutDataTypeStr=uint8  ZeroCross=off
  Constant : Constant  Value=2*pi
  Data Type Duplicate : DataTypeDuplicate
  Flip_0_to_2pi : Subsystem  mask(Flip zero to 2pi){}
      mask help: Flips the inputs into the range zero to +2pi
      mask Help: Flips the inputs into the range zero to +2pi
      mask Display: disp('Flip_0_2pi')
  Switch : Switch  Criteria=u2 ~= 0
  Angle_Flip : Outport
  wires:
  Switch/1 -> Data Type Duplicate/1, Angle_Flip/1
  Add/1 -> Switch/1
  Constant/1 -> Add/1
  Compare To Constant1/1 -> Switch/2
  Flip_0_to_2pi/1(Angle_Flip) -> Add/2, Compare To Constant1/1, Switch/3
  Angle/1 -> Data Type Duplicate/2, Flip_0_to_2pi/1(Angle)

== system Joystick201401023GoldenTriangleLightTEST2/Vicon_Data/Raw Quad Pose from Vicon/Process Vicon Raw Data1/Flip_pi1/Flip_0_to_2pi ==
  Angle : Inport
  Add : Sum
  Compare To Constant1 : simulink/Logic and Bit Operations/Compare To Constant  relop=<  const=0  OutDataTypeStr=uint8  ZeroCross=off
  Constant : Constant  Value=2*pi
  Data Type Duplicate : DataTypeDuplicate
  Flip_2pi : Subsystem  mask(Flip -2pi to 2pi){}
      mask help: Flips the inputs into the range -2pi to +2pi
      mask Help: Flips the inputs into the range -2pi to +2pi
      mask Display: disp('Flip_2pi')
  Switch : Switch  Criteria=u2 ~= 0
  Angle_Flip : Outport
  wires:
  Flip_2pi/1(Angle_Flip) -> Compare To Constant1/1, Add/2, Switch/3
  Compare To Constant1/1 -> Switch/2
  Constant/1 -> Add/1
  Add/1 -> Switch/1
  Angle/1 -> Flip_2pi/1(Angle), Data Type Duplicate/2
  Switch/1 -> Angle_Flip/1, Data Type Duplicate/1

== system Joystick201401023GoldenTriangleLightTEST2/Vicon_Data/Raw Quad Pose from Vicon/Process Vicon Raw Data2/Flip_pi1/Flip_0_to_2pi ==
  Angle : Inport
  Add : Sum
  Compare To Constant1 : simulink/Logic and Bit Operations/Compare To Constant  relop=<  const=0  OutDataTypeStr=uint8  ZeroCross=off
  Constant : Constant  Value=2*pi
  Data Type Duplicate : DataTypeDuplicate
  Flip_2pi : Subsystem  mask(Flip -2pi to 2pi){}
      mask help: Flips the inputs into the range -2pi to +2pi
      mask Help: Flips the inputs into the range -2pi to +2pi
      mask Display: disp('Flip_2pi')
  Switch : Switch  Criteria=u2 ~= 0
  Angle_Flip : Outport
  wires:
  Switch/1 -> Data Type Duplicate/1, Angle_Flip/1
  Angle/1 -> Data Type Duplicate/2, Flip_2pi/1(Angle)
  Add/1 -> Switch/1
  Constant/1 -> Add/1
  Compare To Constant1/1 -> Switch/2
  Flip_2pi/1(Angle_Flip) -> Switch/3, Add/2, Compare To Constant1/1

== system Joystick201401023GoldenTriangleLightTEST2/Vicon_Data/Raw Quad Pose from Vicon/Process Vicon Raw Data3/Flip_pi1/Flip_0_to_2pi ==
  Angle : Inport
  Add : Sum
  Compare To Constant1 : simulink/Logic and Bit Operations/Compare To Constant  relop=<  const=0  OutDataTypeStr=uint8  ZeroCross=off
  Constant : Constant  Value=2*pi
  Data Type Duplicate : DataTypeDuplicate
  Flip_2pi : Subsystem  mask(Flip -2pi to 2pi){}
      mask help: Flips the inputs into the range -2pi to +2pi
      mask Help: Flips the inputs into the range -2pi to +2pi
      mask Display: disp('Flip_2pi')
  Switch : Switch  Criteria=u2 ~= 0
  Angle_Flip : Outport
  wires:
  Flip_2pi/1(Angle_Flip) -> Compare To Constant1/1, Add/2, Switch/3
  Compare To Constant1/1 -> Switch/2
  Constant/1 -> Add/1
  Add/1 -> Switch/1
  Angle/1 -> Flip_2pi/1(Angle), Data Type Duplicate/2
  Switch/1 -> Angle_Flip/1, Data Type Duplicate/1

== system Joystick201401023GoldenTriangleLightTEST2/Vicon_Data/Raw Quad Pose from Vicon/Process Vicon Raw Data7/Flip_pi1/Flip_0_to_2pi ==
  Angle : Inport
  Add : Sum
  Compare To Constant1 : simulink/Logic and Bit Operations/Compare To Constant  relop=<  const=0  OutDataTypeStr=uint8  ZeroCross=off
  Constant : Constant  Value=2*pi
  Data Type Duplicate : DataTypeDuplicate
  Flip_2pi : Subsystem  mask(Flip -2pi to 2pi){}
      mask help: Flips the inputs into the range -2pi to +2pi
      mask Help: Flips the inputs into the range -2pi to +2pi
      mask Display: disp('Flip_2pi')
  Switch : Switch  Criteria=u2 ~= 0
  Angle_Flip : Outport
  wires:
  Switch/1 -> Data Type Duplicate/1, Angle_Flip/1
  Angle/1 -> Data Type Duplicate/2, Flip_2pi/1(Angle)
  Add/1 -> Switch/1
  Constant/1 -> Add/1
  Compare To Constant1/1 -> Switch/2
  Flip_2pi/1(Angle_Flip) -> Switch/3, Add/2, Compare To Constant1/1

== system Joystick201401023GoldenTriangleLightTEST2/Vicon_Data/Raw Quad Pose from Vicon/Process Vicon Raw Data1/Flip_pi1/Flip_0_to_2pi/Flip_2pi ==
  Angle : Inport
  Bias : Bias  Bias=-2*pi
  Constant : Constant  Value=2*pi
  Data Type Duplicate : DataTypeDuplicate
  Modulo : Math  Operator=mod  SaturateOnIntegerOverflow=on
  Sign1 : Signum
  Switch : Switch
  Angle_Flip : Outport
  wires:
  Angle/1 -> Modulo/1, Sign1/1, Data Type Duplicate/1
  Constant/1 -> Modulo/2
  Modulo/1 -> Bias/1, Switch/1
  Sign1/1 -> Switch/2
  Bias/1 -> Switch/3
  Switch/1 -> Angle_Flip/1, Data Type Duplicate/2

== system Joystick201401023GoldenTriangleLightTEST2/Vicon_Data/Raw Quad Pose from Vicon/Process Vicon Raw Data2/Flip_pi1/Flip_0_to_2pi/Flip_2pi ==
  Angle : Inport
  Bias : Bias  Bias=-2*pi
  Constant : Constant  Value=2*pi
  Data Type Duplicate : DataTypeDuplicate
  Modulo : Math  Operator=mod  SaturateOnIntegerOverflow=on
  Sign1 : Signum
  Switch : Switch
  Angle_Flip : Outport
  wires:
  Switch/1 -> Data Type Duplicate/2, Angle_Flip/1
  Bias/1 -> Switch/3
  Sign1/1 -> Switch/2
  Modulo/1 -> Switch/1, Bias/1
  Constant/1 -> Modulo/2
  Angle/1 -> Data Type Duplicate/1, Sign1/1, Modulo/1

== system Joystick201401023GoldenTriangleLightTEST2/Vicon_Data/Raw Quad Pose from Vicon/Process Vicon Raw Data3/Flip_pi1/Flip_0_to_2pi/Flip_2pi ==
  Angle : Inport
  Bias : Bias  Bias=-2*pi
  Constant : Constant  Value=2*pi
  Data Type Duplicate : DataTypeDuplicate
  Modulo : Math  Operator=mod  SaturateOnIntegerOverflow=on
  Sign1 : Signum
  Switch : Switch
  Angle_Flip : Outport
  wires:
  Angle/1 -> Modulo/1, Sign1/1, Data Type Duplicate/1
  Constant/1 -> Modulo/2
  Modulo/1 -> Bias/1, Switch/1
  Sign1/1 -> Switch/2
  Bias/1 -> Switch/3
  Switch/1 -> Angle_Flip/1, Data Type Duplicate/2

== system Joystick201401023GoldenTriangleLightTEST2/Vicon_Data/Raw Quad Pose from Vicon/Process Vicon Raw Data7/Flip_pi1/Flip_0_to_2pi/Flip_2pi ==
  Angle : Inport
  Bias : Bias  Bias=-2*pi
  Constant : Constant  Value=2*pi
  Data Type Duplicate : DataTypeDuplicate
  Modulo : Math  Operator=mod  SaturateOnIntegerOverflow=on
  Sign1 : Signum
  Switch : Switch
  Angle_Flip : Outport
  wires:
  Switch/1 -> Data Type Duplicate/2, Angle_Flip/1
  Bias/1 -> Switch/3
  Sign1/1 -> Switch/2
  Modulo/1 -> Switch/1, Bias/1
  Constant/1 -> Modulo/2
  Angle/1 -> Data Type Duplicate/1, Sign1/1, Modulo/1

== matlab function Joystick201401023GoldenTriangleLightTEST2/Joystick Mapping/check if quad are too close1 ==
  data: u input; ClawPWM output; counter data_store_memory; PWMclaw data_store_memory; JOYtrigger output
function [ClawPWM, JOYtrigger] = CLAW(u)
global counter;
global PWMclaw;
 

if(u~=1)
    if(PWMclaw==1690)
        counter = 1;
        ClawPWM = PWMclaw; 
        JOYtrigger = u;
   
    elseif (PWMclaw==1200)
        counter = 0;
        ClawPWM = PWMclaw;
        JOYtrigger = u;
    end
    
    
else
    if(counter==1)
        PWMclaw = 1200;
        ClawPWM = PWMclaw;
        JOYtrigger = u;
   
    elseif(counter==0)
        PWMclaw = 1690;
        ClawPWM = PWMclaw;
        JOYtrigger = u;
    end
    
end

ClawPWM = PWMclaw;
JOYtrigger = u;
   
end

== stateflow chart Joystick201401023GoldenTriangleLightTEST2/Planning/Trajectory Logic/UAV SF ==
  state AirBorne
    state Game
      state InZone
        state MovetoCenter
          en:
          PosDesired [0]	= 0;
          PosDesired [1]	= 0;
        state ResetJoyHoverAbove
          en:
          PosDesired [2]	= -1.05;
        state Descent
          en:PosDesired [2] = -0.86;
        state Resumeback1
          en:
          PWMclaw 		= 1200;
          JoystickReset	= 1;
          ClawDone 		= 1;
        state CloseClaw1
          en:
          PWM = 1200;
          PosDesired [2] = -0.89;
        state Ascent1
          en:
          PosDesired [2]	 = -1.05;
        (default) -> ResetJoyHoverAbove : {PWM	= 1690;}
        ResetJoyHoverAbove -> MovetoCenter : after (1.3,sec)
        MovetoCenter -> (junction 1476) : after (9,sec)
        (junction 1476) -> Descent : [(abs(Pos[0]-PosDesired[0])<0.01)]
        Descent -> ResetJoyHoverAbove [order 1] : after (4,sec)
        Descent -> CloseClaw1 [order 2] : [Pos[2]>-0.89]
        CloseClaw1 -> Ascent1 : after (1,sec)
        Ascent1 -> Resumeback1 : after (1.1,sec)
      state JoystickCon
        du: PosDesired [0] = Joystick[0];
        PosDesired [1] = Joystick[1];
        PosDesired [2] = Joystick[2];
        PWM 		     = Joystick[3];
        LightPWM	     = 1450;
      state ResetJoyStick1
        en:
        JoystickReset	= 0;
      state Flyaway
        en:
        XFly = TooClose[2];
        YFly = TooClose[3];
        JoystickReset = 1;
        LightPWM 	   = 1250;
      state Fly
        du:
        PosDesired[0] = (XFly-PosDesired[0])*1.4*DeltaT + PosDesired[0];
        PosDesired[1] = (YFly-PosDesired[1])*1.4*DeltaT + PosDesired[1];
      state Fly1
        du:
        PosDesired[0] = (XFly-PosDesired[0])*2.2*DeltaT + PosDesired[0];
        PosDesired[1] = (YFly-PosDesired[1])*2.2*DeltaT + PosDesired[1];
      InZone -> ResetJoyStick1 : [ClawDone ==1]
      JoystickCon -> InZone [order 1] : [(TooClose[1]<=0.45)&&(JoystickTrigger==1)&&(ClawDone == 0)]
      (default) -> ResetJoyStick1
      ResetJoyStick1 -> JoystickCon
      Fly1 -> ResetJoyStick1 : after (1.9,sec)
      Fly -> ResetJoyStick1 : after (1,sec)
      JoystickCon -> Flyaway [order 2] : [TooClose[0]==1]
      Flyaway -> Fly [order 2] : [(TooClose[1]<1.72)||(TooClose[1]>2.45)]
      Flyaway -> Fly1 [order 1] : [(TooClose[1]>=1.72)&&(TooClose[1]<=2.45)]
    state ResetJoyStick
      en:
      JoystickReset = 1;
      PosDesired [3] = 0;
    state TakeOff
      du:HoverThrottle = (H0 - HoverThrottle)*0.25*DeltaT + HoverThrottle ;
      PosDesired[2] = (-1.2- PosDesired[2])*1*DeltaT + PosDesired[2] ;
    state Safety
      state HoverXY1
        en:
        PosDesired 	= Pos;
        PWM 			= 1690;
        LightPWM 		= 1550;
      state HoverZ
        du:PosDesired[2] = (-1.2-PosDesired[2])*0.5*DeltaT + PosDesired[2];
      state ReturnPos1
        du:
        PosDesired[0] = (-1-PosDesired[0])*0.15*DeltaT + PosDesired[0];
        PosDesired[1] = (0-PosDesired[1])*0.15*DeltaT + PosDesired[1];
      state ReturnPos2
        du:
        PosDesired[0] = (1-PosDesired[0])*0.15*DeltaT + PosDesired[0];
        PosDesired[1] = (0-PosDesired[1])*0.15*DeltaT + PosDesired[1];
      state ReturnPos
        du:
        PosDesired[0] = (-1-PosDesired[0])*0.15*DeltaT + PosDesired[0];
        PosDesired[1] = (3.3-PosDesired[1])*0.15*DeltaT + PosDesired[1];
      state Descent2
        du: PosDesired[2] = (-0.2-PosDesired[2])*0.5*DeltaT + PosDesired[2];
      (default) -> HoverXY1
      HoverXY1 -> HoverZ
      HoverZ -> (junction 1500) : [abs(Pos[2]+1.3)<0.15]
      (junction 1500) -> (junction 1467) : [Q2[2]<-2.97]
      (junction 1467) -> ReturnPos1 [order 3] : [(abs(Pos[0])<=0)&&(abs(Pos[1])<0)]
      (junction 1467) -> ReturnPos2 [order 1] : [(abs(Pos[0])>0)&&(abs(Pos[1])<0)]
      (junction 1467) -> ReturnPos [order 2] : [abs(Pos[1])>=0]
      ReturnPos1 -> ReturnPos : [(abs(Pos[0]+1)+abs(Pos[1]))<0.2]
      ReturnPos2 -> ReturnPos : [(abs(Pos[0]-1)+abs(Pos[1]))<0.2]
      ReturnPos -> Descent2 : [(abs(Pos[0]+1)+abs(Pos[1]-3.3))<0.4]
    (default) -> TakeOff : {PosDesired = Pos;}
    TakeOff -> ResetJoyStick : [abs(Q2[0]-2)<0.2]
    ResetJoyStick -> Game
    Game -> Safety [order 3] : [RC[5] > 0]
    Game -> Safety [order 1] : after (88.5,sec)
    Game -> Safety [order 2] : [Q2[2]<-2.97]
  note: Joystick[x]:
      |
      | 0. X-axis
      | 1. Y-axis
      | 2. Z-Axis
      | 3. PWM
      |
      | Joystick Trigger = Trigger state
      |
      |
      | TooClose[x]:
      |
      | Where x=:
      | 0.	Bound
      | 1.	Q5 Current Radius
      | 2.	X
      | 3.	Y
  state Landing
    state Descending
      en:PosDesired = Pos;
      du:PosDesired[2] = (0.2- PosDesired[2])*1*DeltaT + PosDesired[2] ;
    state CutThrottle
      en: PWM=1600;
      du:HoverThrottle = (0.0- HoverThrottle)*3*DeltaT + HoverThrottle ;
    (default) -> Descending
    Descending -> CutThrottle : [Pos[2] >(0.0 -0.2)]
  Landing -> AirBorne : [RC[6] > 0.5]
  AirBorne -> Landing : [RC[6] < -0.5]
  (default) -> Landing : {HoverThrottle = 0;}
  data: PosDesired output double size=4; HoverThrottle output double size=1; RC input size=8; Pos input size=4; DeltaT parameter size=1; H0 parameter size=1; Kl parameter size=1; VelCmd local double size=2 =0; PWM output double; PI parameter size=1; Joystick input; TooClose input double; JoystickReset output double size=1; XFly local double size=1; YFly local double size=1; PWMclaw data_store_memory size=1; JoystickTrigger input boolean size=1; ClawDone local boolean =0; LightPWM data_store_memory; Q2 input double
